simulink model "Vehicle"  (R2024b)
settings: Solver=ode4  StartTime=0.0  StopTime=inf  FixedStep=vehicleParams.Ts  RelTol=1e-3
PreLoadFcn:
  | % Load scenario parameters if not already loaded
  | if ~exist('hostParams', 'var')
  |     hostParams = helperScenarioParams;
  | end
  | 
  | % Load vehicle parameters if not already loaded
  | if ~exist('vehicleParams', 'var')
  |     vehicleParams = helperVehicleParams;
  | end
  | 
  | % Load PathFollower parameters if not already loaded
  | if ~exist('controllerParams', 'var')
  |     controllerParams = helperPathFollowerParams;
  | end
  | 
  | % Set IP addresses to local computer if they are not provided
  | if ~exist('ipAddress', 'var')
  |     ipAddress = helperIPAddresses;
  | end
libraries: slrealtimeiplib x3, slrealtimeutilitieslib x2, simulink x1, autolibshared x1
settings Model: SimulationMode=external  ExtModeTrigDuration=100000  Creator=smaddina  LastModifiedBy=demo-user2
settings SolverCC: ConcurrentTasks=on  PositivePriorityOrder=on
settings OptimizationCC: BlockReduction=off  OptimizeBlockIOStorage=off
settings DebuggingCC: TasksWithSamePriorityMsg=none
settings HardwareCC: ProdBitPerLong=64  ProdLongLongMode=on  ProdHWDeviceType=Intel->x86-64 (Linux 64)
settings RTWCC: Description=Speedgoat Real-Time Target Machine  SystemTargetFile=speedgoat.tlc  TemplateMakefile=slrealtime_default_tmf  Toolchain=Simulink Real-Time Toolchain  BuildConfiguration=Faster Runs  CodeExecutionProfiling=on  TargetLang=C++
settings CodeAppCC: MaxIdLength=95
settings SimulinkRealTimeTargetCC: InstructionSetFMA=off  LogToMDFFile=off

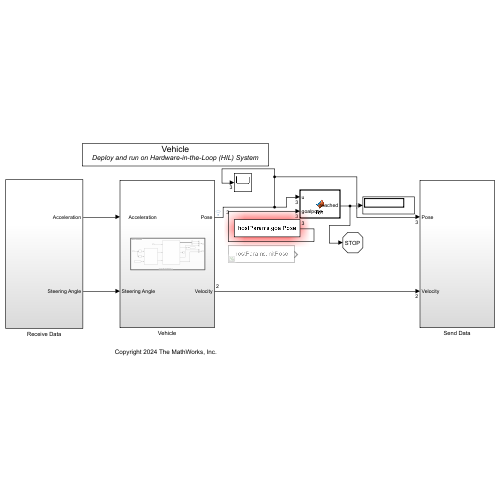
[thumbnail: Simulink's stored preview of the top-level diagram]
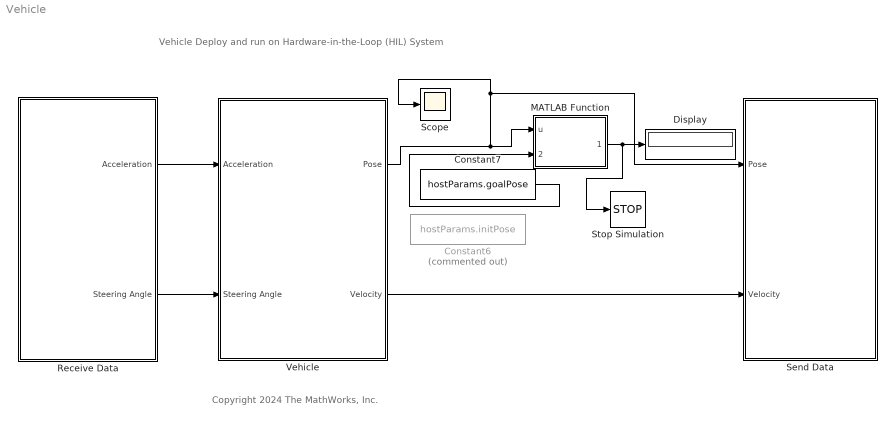
== system Vehicle ==
  note: Vehicle
      | Deploy and run on Hardware-in-the-Loop (HIL) System
  note: Copyright 2024 The MathWorks, Inc.
  Constant6 : Constant  Commented=on  Value=hostParams.initPose
  Constant7 : Constant  Value=hostParams.goalPose
  Display : Display
  MATLAB Function : MATLAB Function  TreatAsAtomicUnit=on
  Receive Data : Subsystem
  Scope : Scope
  Send Data : Subsystem
  Stop Simulation : Stop
  Vehicle : Subsystem
  wires:
  Vehicle/1(" Pose") -> MATLAB Function/1(u), Send Data/1(Pose), Scope/1
  Vehicle/2(Velocity) -> Send Data/2(Velocity)
  Receive Data/2(Steering Angle) -> Vehicle/2(Steering Angle)
  Receive Data/1(Acceleration) -> Vehicle/1("     Acceleration")
  Constant7/1 -> MATLAB Function/2(goalpose)
  MATLAB Function/1(reached) -> Stop Simulation/1, Display/1

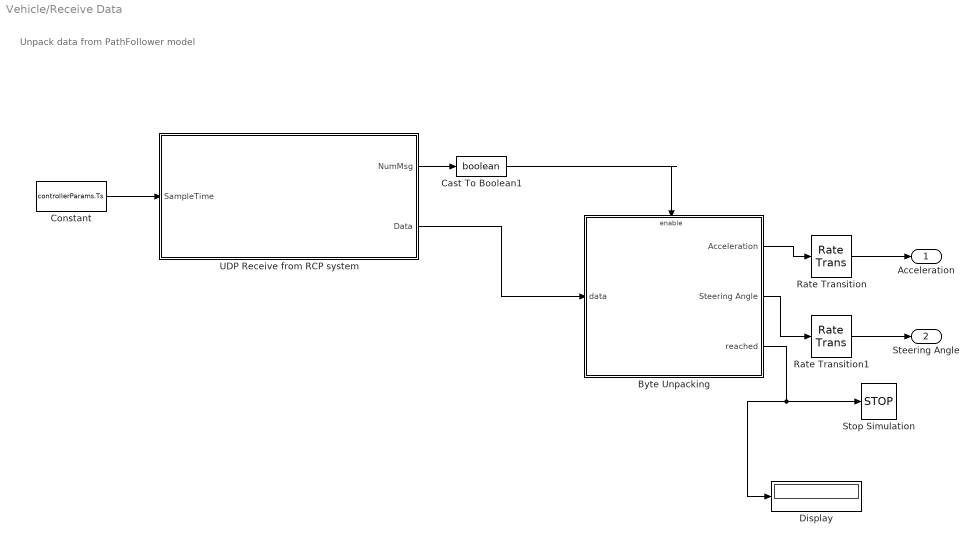
== system Vehicle/Receive Data ==
  note: Unpack data from PathFollower model
  Byte Unpacking : Subsystem  TreatAsAtomicUnit=on
  Cast To Boolean1 : DataTypeConversion  OutDataTypeStr=boolean  SaturateOnIntegerOverflow=off  RndMeth=Floor
  Constant : Constant  Value=controllerParams.Ts  SampleTime=controllerParams.Ts
  Display : Display
  Rate Transition : RateTransition
  Rate Transition1 : RateTransition
  Stop Simulation : Stop
  UDP Receive from RCP system : Subsystem  TreatAsAtomicUnit=on
  Acceleration : Outport
  Steering Angle : Outport  Port=2
  wires:
  Byte Unpacking/2(Steering Angle) -> Rate Transition1/1
  Cast To Boolean1/1 -> Byte Unpacking/Enable
  Byte Unpacking/1(Acceleration) -> Rate Transition/1
  Rate Transition/1 -> Acceleration/1
  Rate Transition1/1 -> Steering Angle/1
  Constant/1 -> UDP Receive from RCP system/1(SampleTime)
  UDP Receive from RCP system/1(NumMsg) -> Cast To Boolean1/1
  UDP Receive from RCP system/2(Data) -> Byte Unpacking/1(data)
  Byte Unpacking/3(reached) -> Stop Simulation/1, Display/1

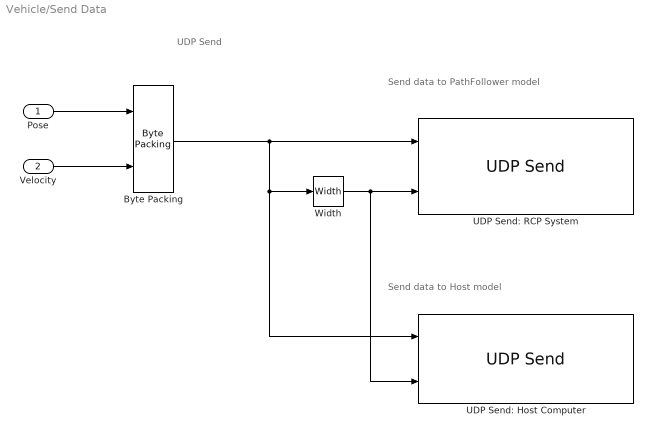
== system Vehicle/Send Data ==
  note: Send data to Host model
  note: Send data to PathFollower model
  note: UDP Send
  Pose : Inport
  Velocity : Inport  Port=2
  Byte Packing : slrealtimeutilitieslib/Byte Packing  MaskPackedDataType=uint8  MaskUnpackedDataTypes={'double', 'double'}  MaskAlignment=1
  UDP Send: Host Computer : slrealtimeiplib/UDP Send  useHostTargetConn=on  toAddress=ipAddress.hostSystem  toPort=8005  sampleTime=-1  enableMessage=off  ipAddress=hostIP  localPort=-1
  UDP Send: RCP System : slrealtimeiplib/UDP Send  useHostTargetConn=on  toAddress=ipAddress.rcpSystem  toPort=8002  sampleTime=-1  enableMessage=off  localPort=-1
  Width : Width
  wires:
  Width/1 -> UDP Send: Host Computer/2, UDP Send: RCP System/2
  Byte Packing/1 -> UDP Send: Host Computer/1, Width/1, UDP Send: RCP System/1
  Pose/1 -> Byte Packing/1
  Velocity/1 -> Byte Packing/2

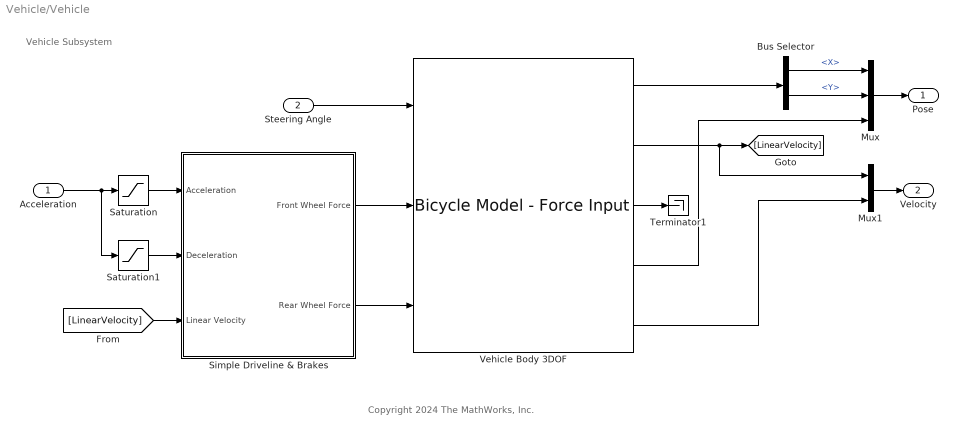
== system Vehicle/Vehicle ==
  note: Vehicle Subsystem
  note: Copyright 2024 The MathWorks, Inc.
  "     Acceleration" : Inport  Unit=m/s
  Steering Angle : Inport  Port=2
  Bus Selector : BusSelector  OutputSignals=InertFrm.Cg.Disp.X,InertFrm.Cg.Disp.Y
  Mux : Mux  Inputs=3
  Mux1 : Mux  Inputs=2
  Saturation : Saturate  UpperLimit=inf  LowerLimit=0
  Saturation1 : Saturate  UpperLimit=0  LowerLimit=-inf
  Simple Driveline & Brakes : Subsystem
  Terminator1 : Terminator
  Vehicle Body 3DOF : autolibshared/Bicycle Model - Force Input  trackMode=Single (bicycle)  inputMode=External longitudinal forces  frontSteerMode=on  rearSteerMode=off  windMode=off  muMode=off  extFMode=off  extMMode=off  aMode=2  NF=vehicleParams.numWheelsFront  NR=vehicleParams.numWheelsRear  m=vehicleParams.mass  a=vehicleParams.lengthCGToFrontAxle  b=vehicleParams.lengthCGToRearAxle  h=vehicleParams.heightCG  X_o=hostParams.initPose(1)  xdot_o=0  CalphaMode=off  sigmaMode=on  w=[1.4,1.4]  Cy_f=vehicleParams.corneringStiffnessFrontTire  Cy_r=vehicleParams.corneringStiffnessRearTire  sigma_f=.1  sigma_r=.1  alpha_f_brk=[-.1 .1]  Cy_f_data=[-9e3 9e3]  alpha_r_brk=[-.1 .1]  Cy_r_data=[-9e3 9e3]  Y_o=hostParams.initPose(2)  ydot_o=0  Izz=vehicleParams.yawInertia  psi_o=hostParams.initPose(3)  r_o=0  Af=2  Cd=.3  Cl=.1  Cpm=.1  beta_w=[0 0.01:0.01:0.3]  Cs=[0 0.01:0.01:0.3]  Cym=[0 1e-6:0.01:0.3]  Pabs=101325  Tair=273  g=9.81  mu=1  xdot_tol=.01  Fznom=5000  Fxtire_sat=1e6  Fytire_sat=1e6  longOff=0  latOff=0  vertOff=0
      settings: LibrarySourceBlock=vehdynlibeom/Bicycle Model - Force Input
  " Pose" : Outport  VectorParamsAs1DForOutWhenUnconnected=off
  Velocity : Outport  Port=2  VectorParamsAs1DForOutWhenUnconnected=off
  wires:
  Mux1/1 -> Velocity/1
  Vehicle Body 3DOF/5 -> Mux1/2
  "     Acceleration"/1 -> Saturation1/1, Saturation/1
  Vehicle Body 3DOF/1 -> Bus Selector/1
  Bus Selector/2 -> Mux/2  "<Y>"
  Vehicle Body 3DOF/4 -> Mux/3
  Bus Selector/1 -> Mux/1  "<X>"
  Mux/1 -> " Pose"/1
  Vehicle Body 3DOF/3 -> Terminator1/1
  Vehicle Body 3DOF/2 -> [LinearVelocity], Mux1/1
  Simple Driveline & Brakes/2(Rear Wheel Force) -> Vehicle Body 3DOF/3
  Saturation/1 -> Simple Driveline & Brakes/1(Acceleration)
  Saturation1/1 -> Simple Driveline & Brakes/2(Deceleration)
  [LinearVelocity] -> Simple Driveline & Brakes/3(Linear Velocity)
  Steering Angle/1 -> Vehicle Body 3DOF/1
  Simple Driveline & Brakes/1(Front Wheel Force) -> Vehicle Body 3DOF/2

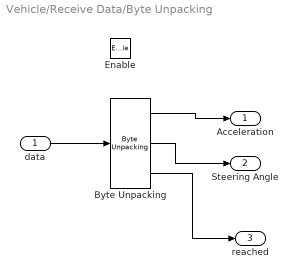
== system Vehicle/Receive Data/Byte Unpacking ==
  data : Inport
  Enable : EnablePort
  Byte Unpacking : slrealtimeutilitieslib/Byte Unpacking  MaskUnpackedDataTypes="{ 'double',  'double','boolean'}"  MaskUnpackedDataSizes={[1],[1],[1]}  MaskAlignment=1
  Acceleration : Outport
  Steering Angle : Outport  Port=2
  reached : Outport  Port=3
  wires:
  Byte Unpacking/1 -> Acceleration/1
  Byte Unpacking/2 -> Steering Angle/1
  data/1 -> Byte Unpacking/1
  Byte Unpacking/3 -> reached/1

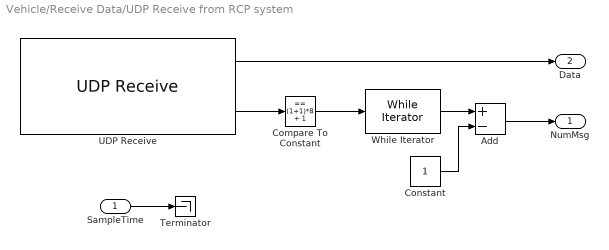
== system Vehicle/Receive Data/UDP Receive from RCP system ==
  SampleTime : Inport
  Add : Sum  Inputs=+-
  Compare To Constant : simulink/Logic and Bit Operations/Compare To Constant  relop===  const=(1+1)*8 + 1  OutDataTypeStr=boolean
  Constant : Constant
  Terminator : Terminator
  UDP Receive : slrealtimeiplib/UDP Receive  useHostTargetConn=on  ipAddress=10.10.10.15  localPort=8003  rcvWidth=(1+1)*8 +1  rcvFmAny=on  fmAddress='10.10.10.10'  sampleTime=-1  enableMessage=off  maxPackets=1
  While Iterator : WhileIterator  WhileBlockType=do-while  ShowIterationPort=on
  NumMsg : Outport
  Data : Outport  Port=2
  wires:
  Compare To Constant/1 -> While Iterator/1
  UDP Receive/1 -> Data/1
  UDP Receive/2 -> Compare To Constant/1
  Add/1 -> NumMsg/1
  While Iterator/1 -> Add/1
  Constant/1 -> Add/2
  SampleTime/1 -> Terminator/1

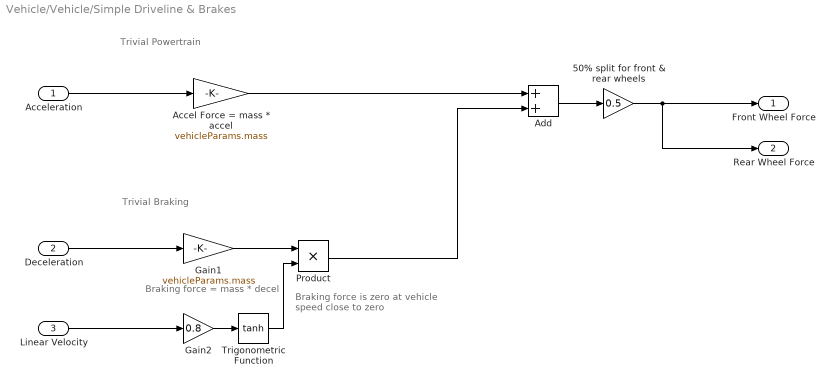
== system Vehicle/Vehicle/Simple Driveline & Brakes ==
  note: Braking force = mass * decel
  note: Trivial Powertrain
  note: Trivial Braking
  note: Braking force is zero
      | at vehicle speed close
      | to zero
  Acceleration : Inport
  Deceleration : Inport  Port=2
  Linear Velocity : Inport  Port=3
  50% split for front & rear wheels : Gain  Gain=0.5
  Accel Force = mass * accel : Gain  Gain=vehicleParams.mass
  Add : Sum
  Gain1 : Gain  Gain=vehicleParams.mass
  Gain2 : Gain  Gain=0.8
  Product : Product
  Trigonometric Function : Trigonometry  Operator=tanh
  Front Wheel Force : Outport
  Rear Wheel Force : Outport  Port=2
  wires:
  Acceleration/1 -> Accel Force = mass * accel/1
  Deceleration/1 -> Gain1/1
  Linear Velocity/1 -> Gain2/1
  Gain2/1 -> Trigonometric Function/1
  Gain1/1 -> Product/1
  Trigonometric Function/1 -> Product/2
  Add/1 -> 50% split for front & rear wheels/1
  50% split for front & rear wheels/1 -> Front Wheel Force/1, Rear Wheel Force/1
  Product/1 -> Add/2
  Accel Force = mass * accel/1 -> Add/1

== matlab function Vehicle/MATLAB Function ==
  data: u input; reached output; goalpose input
function reached = fcn(u, goalpose)
%#codegen

distance = sqrt((u([1])-goalpose([1]))^2 +(u([2])-goalpose([2]))^2 );
if distance<=5
    reached = true;
else

   reached = false;
end
% velgain = 1;
% pose = u;
end
